simulink model "OHC_Lowpass_Filter"  (R2019b)
settings: Solver=VariableStepAuto  StartTime=0.0  StopTime=testtime  RelTol=1e-3
InitFcn:
  | OHC_Lowpass_Test_Parameters
StopFcn:
  | Verify_OHC_Lowpass_Filter
undefined symbols (not defined in the file or in its folder): c1LPohc, c2LPohc, dfilt, Fs, gainohc, OHCLPcoeffs
libraries: dsparch4 x2, dspsrcs4 x2
settings Model: Creator=mblun
settings OptimizationCC: BlockReduction=off  ConditionallyExecuteInputs=off  DefaultParameterBehavior=Inlined
settings DebuggingCC: AlgebraicLoopMsg=error
settings HardwareCC: ProdBitPerPointer=32  ProdBitPerSizeT=32  ProdBitPerPtrDiffT=32  ProdLargestAtomicFloat=None  ProdIntDivRoundTo=Undefined  ProdEndianess=Unspecified  ProdWordSize=32  ProdHWDeviceType=ASIC/FPGA->ASIC/FPGA  TargetBitPerPointer=64  TargetBitPerSizeT=64  TargetBitPerPtrDiffT=64  TargetLongLongMode=on  TargetIntDivRoundTo=Zero  TargetEndianess=LittleEndian  TargetWordSize=64  TargetHWDeviceType=Custom Processor->MATLAB Host Computer  ProdEqTarget=off
settings SFSimCC: CustomCodeUndefinedFunction=UseInterfaceOnly

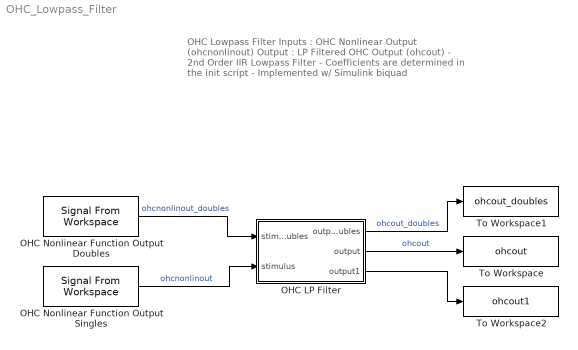
== system OHC_Lowpass_Filter ==
  note: OHC Lowpass Filter
      |
      | Inputs : OHC Nonlinear Output (ohcnonlinout)
      |
      | Output : LP Filtered OHC Output (ohcout)
      |
      | - 2nd Order IIR Lowpass Filter
      |
      | - Coefficients are determined in the init script
      |
      | - Implemented w/ Simulink biquad
  OHC LP Filter : Subsystem
  OHC Nonlinear Function Output Doubles : dspsrcs4/Signal From Workspace  X=RxSignal_doubles  Ts=1/Fs  nsamps=1  OutputAfterFinalValue=Setting to zero  ignoreOrWarnInputAndFrameLengths=off  OutputFrames=off
  OHC Nonlinear Function Output Singles : dspsrcs4/Signal From Workspace  X=RxSignal  Ts=1/Fs  nsamps=1  OutputAfterFinalValue=Setting to zero  ignoreOrWarnInputAndFrameLengths=off  OutputFrames=off
  To Workspace : ToWorkspace  VariableName=ohcout  SampleTime=-1
      settings: Save2DSignal=2-D array (concatenate along first dimension)
  To Workspace1 : ToWorkspace  VariableName=ohcout_doubles  SampleTime=-1
      settings: Save2DSignal=2-D array (concatenate along first dimension)
  To Workspace2 : ToWorkspace  VariableName=ohcout1  SampleTime=-1
      settings: Save2DSignal=2-D array (concatenate along first dimension)
  wires:
  OHC Nonlinear Function Output Singles/1 -> OHC LP Filter/2(stimulus)  "ohcnonlinout"
  OHC LP Filter/2(output) -> To Workspace/1  "ohcout"
  OHC Nonlinear Function Output Doubles/1 -> OHC LP Filter/1(stimulus_doubles)  "ohcnonlinout_doubles"
  OHC LP Filter/1(output_doubles) -> To Workspace1/1  "ohcout_doubles"
  OHC LP Filter/3(output1) -> To Workspace2/1

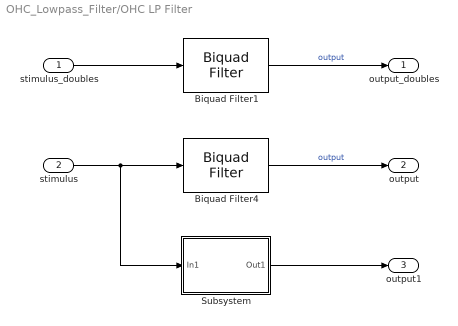
== system OHC_Lowpass_Filter/OHC LP Filter ==
  stimulus_doubles : Inport
  stimulus : Inport  Port=2
  Biquad Filter1 : dsparch4/Biquad Filter  FilterSource=Dialog parameters  CoeffSource=Specify via dialog  FilterObject=dfilt.df2tsos([1 0.3 0.4],[1 0.1 0.2])  IIRFiltStruct=Direct form I  BiQuadCoeffs=[gainohc*c2LPohc gainohc*c2LPohc 0 1 -c1LPohc 0; gainohc*c2LPohc gainohc*c2LPohc 0 1 -c1LPohc 0]  ScaleValues=1  IC=0  ICnum=0  ICden=0  a0Flag=Warning  optimizeScaleValues=on  ScaleValueMode=Specify via input port (g)  roundingMode=Floor  overflowMode=on  scaleValueFracLength=14  denProdOutputFracLength=30  denAccumFracLength=30  secondMemoryFracLength=15
      settings: SourceProductName=DSP System Toolbox
  Biquad Filter4 : dsparch4/Biquad Filter  FilterSource=Dialog parameters  CoeffSource=Specify via dialog  FilterObject=dfilt.df2tsos([1 0.3 0.4],[1 0.1 0.2])  IIRFiltStruct=Direct form I  BiQuadCoeffs=OHCLPcoeffs  ScaleValues=1  IC=0  ICnum=0  ICden=0  a0Flag=Warning  optimizeScaleValues=on  ScaleValueMode=Specify via input port (g)  roundingMode=Floor  overflowMode=on  scaleValueFracLength=14  denProdOutputFracLength=30  denAccumFracLength=30  secondMemoryFracLength=15
      settings: SourceProductName=DSP System Toolbox
  Subsystem : Subsystem
  output_doubles : Outport  VectorParamsAs1DForOutWhenUnconnected=off
  output : Outport  Port=2  VectorParamsAs1DForOutWhenUnconnected=off
  output1 : Outport  Port=3  VectorParamsAs1DForOutWhenUnconnected=off
  wires:
  stimulus/1 -> Subsystem/1(In1), Biquad Filter4/1
  Biquad Filter4/1 -> output/1  "output"
  Biquad Filter1/1 -> output_doubles/1  "output"
  stimulus_doubles/1 -> Biquad Filter1/1
  Subsystem/1(Out1) -> output1/1

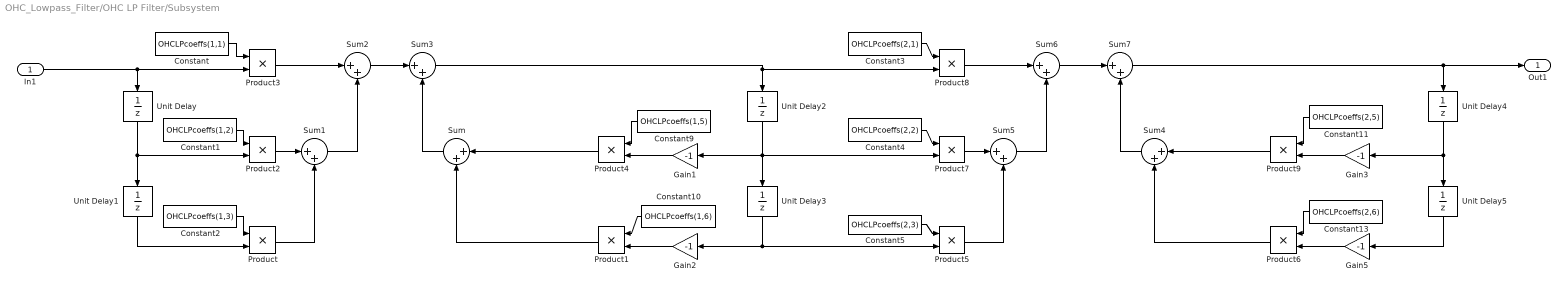
== system OHC_Lowpass_Filter/OHC LP Filter/Subsystem ==
  In1 : Inport
  Constant : Constant  Value=OHCLPcoeffs(1,1)  OutDataTypeStr=single  SampleTime=-1
  Constant1 : Constant  Value=OHCLPcoeffs(1,2)  OutDataTypeStr=single  SampleTime=-1
  Constant10 : Constant  Value=OHCLPcoeffs(1,6)  OutDataTypeStr=single  SampleTime=-1
  Constant11 : Constant  Value=OHCLPcoeffs(2,5)  OutDataTypeStr=single  SampleTime=-1
  Constant13 : Constant  Value=OHCLPcoeffs(2,6)  OutDataTypeStr=single  SampleTime=-1
  Constant2 : Constant  Value=OHCLPcoeffs(1,3)  OutDataTypeStr=single  SampleTime=-1
  Constant3 : Constant  Value=OHCLPcoeffs(2,1)  OutDataTypeStr=single  SampleTime=-1
  Constant4 : Constant  Value=OHCLPcoeffs(2,2)  OutDataTypeStr=single  SampleTime=-1
  Constant5 : Constant  Value=OHCLPcoeffs(2,3)  OutDataTypeStr=single  SampleTime=-1
  Constant9 : Constant  Value=OHCLPcoeffs(1,5)  OutDataTypeStr=single  SampleTime=-1
  Gain{1..3,5} (4 alike) : Gain  Gain=-1
  Product{,1..9} (10 alike) : Product
  Sum{,1..7} (8 alike) : Sum  Inputs=|++
  Unit Delay{,1..5} (6 alike) : UnitDelay  SampleTime=-1  HasFrameUpgradeWarning=on
  Out1 : Outport
  wires:
  Constant2/1 -> Product/1
  Unit Delay/1 -> Unit Delay1/1, Product2/2
  Sum1/1 -> Sum2/2
  Constant3/1 -> Product8/1
  Constant13/1 -> Product6/1
  Constant/1 -> Product3/1
  Constant1/1 -> Product2/1
  Constant9/1 -> Product4/1
  Unit Delay2/1 -> Product7/2, Unit Delay3/1, Gain1/1
  In1/1 -> Product3/2, Unit Delay/1
  Sum5/1 -> Sum6/2
  Constant10/1 -> Product1/1
  Unit Delay4/1 -> Unit Delay5/1, Gain3/1
  Product7/1 -> Sum5/1
  Gain1/1 -> Product4/2
  Constant4/1 -> Product7/1
  Product3/1 -> Sum2/1
  Product2/1 -> Sum1/1
  Product5/1 -> Sum5/2
  Constant5/1 -> Product5/1
  Unit Delay3/1 -> Product5/2, Gain2/1
  Unit Delay1/1 -> Product/2
  Unit Delay5/1 -> Gain5/1
  Product8/1 -> Sum6/1
  Gain2/1 -> Product1/2
  Gain3/1 -> Product9/2
  Gain5/1 -> Product6/2
  Constant11/1 -> Product9/1
  Product/1 -> Sum1/2
  Sum2/1 -> Sum3/1
  Sum6/1 -> Sum7/1
  Product4/1 -> Sum/1
  Product1/1 -> Sum/2
  Product9/1 -> Sum4/1
  Product6/1 -> Sum4/2
  Sum/1 -> Sum3/2
  Sum3/1 -> Product8/2, Unit Delay2/1
  Sum4/1 -> Sum7/2
  Sum7/1 -> Unit Delay4/1, Out1/1
